simulink model "model"  (R2024b)
settings: Solver=ode1  StartTime=0.0  StopTime=10  FixedStep=0.0001  RelTol=1e-3
values from neighbouring files (symbols this model uses):
  a1 = c*a2    (= 810)    [init.m]
  a2 = c*a3    (= 270)    [init.m]
  a3 = c*a4    (= 90)    [init.m]
  a4 = c*10    (= 30)    [init.m]
  c1 = 50    [init.m]
  c2 = 1    [init.m]
  d = 100    [init.m]
  dis_gain = 30    [init.m]
  epsilon = 1    [init.m]
  i = 20    [init.m]
  k = 5    [init.m]
  mu = 0.9    [init.m]
  p = 400    [init.m]
  phi_frist = 0    [init.m]
  psi_frist = 0    [init.m]
  tau_p_max = 3000000    [init.m]
  theta_frist = 0    [init.m]
  umax = pi/2 - 0.01    (= 1.56079632679)    [init.m]
  w = wo    (= 50)    [init.m]
  wo = 50    [init.m]
  x_frist = 0    [init.m]
  y_frist = 0    [init.m]
  z_frist = 0    [init.m]
libraries: fod x36, slpidlib x6, simulink x1
(part 3 of 4)

== matlab function model/FO_SMC_ESO/Subsystem2/线性反馈 ==
  data: eta input; tau_1 output size=6; deta input; nu input; M_eta output; J output; J_inv output
function [tau_1,M_eta,J,J_inv] = fcn(eta,deta,nu)

m = 5.5;
    I_x = 0.12;
    I_y = 0.25;
    I_z = 0.2;
    V = m;
    g = 9.8;

    x_B = 0;
    y_B = 0;
    z_B = -0.01;

    X_du = -2.61;
    K_dp = -0.15;
    X_u = -2.47;
    K_P = -0.82;
    X_uu = -8.33;
    K_pp = -2.95;
    Y_dv = -5.56;
    M_dq = -0.26;
    Y_v = -3.54;
    M_q = -0.9;
    Y_vv = -10.82;
    M_qq = -3.687;
    Z_dw = -9.75;
    N_dr = -0.21;
    Z_w = -2.38;
    N_r = -0.45;
    Z_ww = -14.13;
    N_rr = -1.56;

    m_u = m - X_du;
    m_v = m - Y_dv;
    m_w = m - Z_dw;
    m_p = I_x - K_dp;
    m_q = I_y - M_dq;
    m_r = I_z - N_dr;

    m_u = m - X_du;
    m_v = m - Y_dv;
    m_w = m - Z_dw;
    m_p = I_x - K_dp;
    m_q = I_y - M_dq;
    m_r = I_z - N_dr;

    x = eta(1);
    y = eta(2);
    z = eta(3);
    phi = eta(4);
    theta = eta(5);
    psi = eta(6);

    J =  [cos(psi)*cos(theta) -sin(psi)*cos(phi)+sin(phi)*sin(theta)*cos(psi) sin(psi)*sin(phi)+sin(theta)*cos(psi)*cos(phi) 0 0 0;
         sin(psi)*cos(theta) cos(psi)*cos(phi)+sin(phi)*sin(theta)*sin(psi) -cos(psi)*sin(phi)+sin(theta)*sin(psi)*cos(phi) 0 0 0;
         -sin(theta) sin(phi)*cos(theta) cos(psi)*cos(theta) 0 0 0;
         0 0 0 1 sin(phi)*tan(theta) cos(phi)*tan(theta);
         0 0 0 0 cos(phi) -sin(phi);
         0 0 0 0 sin(phi)/cos(theta) cos(phi)/cos(theta)];

    J_inv = inv(J);

    u = nu(1);
    v = nu(2);
    w = nu(3);
    p = nu(4);
    q = nu(5);
    r = nu(6);

    
    dphi = deta(4);
    dtheta = deta(5);
    dpsi = deta(6);

    M = [m_u 0 0 0 0 0;
         0 m_v 0 0 0 0;
         0 0 m_w 0 0 0;
         0 0 0 m_p 0 0;
         0 0 0 0 m_q 0;
         0 0 0 0 0 m_r];

    C = [0 0 0 0 m_w*w -m_r*v;
         0 0 0 -m_w*w 0 m_u*u;
         0 0 0 m_v*v -m_u*u 0;
         0 m_w*w -m_v*v 0 m_r*r -m_q*q;
         -m_w*w 0 m_u*u -m_r*r 0 m_p*p;
         m_v*v -m_u*u 0 m_q*q -m_p*p 0];
    
    D = -[X_uu*abs(u) 0 0 0 0 0;
          0 Y_vv*abs(v) 0 0 0 0;
          0 0 Z_ww*abs(w) 0 0 0;
          0 0 0 K_pp*abs(p) 0 0;
          0 0 0 0 M_qq*abs(q) 0;
          0 0 0 0 0 N_rr*abs(r)];
    dJ = [
        % 第一行
        -sin(psi)*cos(theta)*dpsi - cos(psi)*sin(theta)*dtheta, ...
        (-cos(psi)*cos(phi) - sin(phi)*sin(theta)*sin(psi))*dpsi + ...
        (sin(phi)*cos(theta)*cos(psi))*dtheta + ...
        (sin(psi)*sin(phi) + cos(phi)*sin(theta)*cos(psi))*dphi, ...
        (cos(psi)*sin(phi) - sin(theta)*sin(psi)*cos(phi))*dpsi + ...
        (cos(psi)*cos(phi)*cos(theta))*dtheta + ...
        (sin(psi)*cos(phi) - sin(theta)*cos(psi)*sin(phi))*dphi, ...
        0, 0, 0;
        
        % 第二行
        cos(psi)*cos(theta)*dpsi - sin(psi)*sin(theta)*dtheta, ...
        (-sin(psi)*cos(phi) + sin(phi)*sin(theta)*cos(psi))*dpsi + ...
        (sin(phi)*cos(theta)*sin(psi))*dtheta + ...
        (-cos(psi)*sin(phi) + cos(phi)*sin(theta)*sin(psi))*dphi, ...
        (sin(psi)*sin(phi) + sin(theta)*cos(psi)*cos(phi))*dpsi + ...
        (sin(psi)*cos(phi)*cos(theta))*dtheta + ...
        (-cos(psi)*cos(phi) - sin(theta)*sin(psi)*sin(phi))*dphi, ...
        0, 0, 0;
        
        % 第三行
        -cos(theta)*dtheta, ...
        cos(phi)*cos(theta)*dphi - sin(phi)*sin(theta)*dtheta, ...
        -sin(psi)*cos(theta)*dpsi - cos(psi)*sin(theta)*dtheta, ...
        0, 0, 0;
        
        % 第四行
        0, 0, 0, ...
        0, ...
        cos(phi)*tan(theta)*dphi + sin(phi)*(1/cos(theta)^2)*dtheta, ...
        -sin(phi)*tan(theta)*dphi + cos(phi)*(1/cos(theta)^2)*dtheta;
        
        % 第五行
        0, 0, 0, ...
        0, ...
        -sin(phi)*dphi, ...
        -cos(phi)*dphi;
        
        % 第六行
        0, 0, 0, ...
        0, ...
        cos(phi)*(1/cos(theta))*dphi + sin(phi)*(sin(theta)/cos(theta)^2)*dtheta, ...
        -sin(phi)*(1/cos(theta))*dphi + cos(phi)*(sin(theta)/cos(theta)^2)*dtheta
    ];
    
    B = g*V;

    g_eta = [0;0;0;-z_B*B*cos(theta)*sin(phi);-z_B*B*sin(theta);0];

    M_eta = J_inv'*M*J_inv;
    C_eta = J_inv'*(C-M*J_inv*dJ)*J_inv;
    G_eta = J_inv'*g_eta;
    D_eta = J_inv'*D*J_inv;

tau_1 = J'*(C_eta*deta+D_eta*deta+G_eta);

== matlab function model/FO_SMC_ESO/LESO/Subsystem1/Subsystem6/MATLAB Function2 ==
  data: h input; dh output size=3; eta input; tau_0 input; wo input
function dh = fcn(h,eta,tau_0,wo)

e = eta-h(1);

b1 = 3*wo;
b2  = 3*wo^2;
b3 = wo^3;

dh = [h(2)+b1*e;
    h(3)+b2*e+tau_0;
    b3*e;
    ];

== matlab function model/tau_d/MATLAB Function ==
  data: t input; y output
function y = fcn(t)
    
y = [3*sin(t)*cos(t);3*sin(t)*cos(t);3*sin(t)*cos(t)];

== matlab function model/tau_d/MATLAB Function1 ==
  data: t input; y output
function y = fcn(t)
    
y = [3*sin(t)*cos(t);3*sin(t)*cos(t);3*sin(t)*cos(t)];

== matlab function model/FO_SMC_ESO/LESO/MATLAB Function3 ==
  data: M_eta input; tau_0 output; J_inv input; tau_c input
function tau_0 = fcn(M_eta,J_inv,tau_c)

tau_0 = inv(M_eta)*J_inv'*tau_c;

== matlab function model/FO_SMC_ESO/LESO/MATLAB Function4 ==
  data: J input; tau_2 output; M_eta input; h3 input
function tau_2 = fcn(J,M_eta,h3)

tau_2 = -J'*M_eta*h3;

== matlab function model/FO_SMC_ESO/LESO/Subsystem1/Subsystem1/MATLAB Function2 ==
  data: h input; dh output size=3; eta input; tau_0 input; wo input
function dh = fcn(h,eta,tau_0,wo)

e = eta-h(1);

b1 = 3*wo;
b2  = 3*wo^2;
b3 = wo^3;

dh = [h(2)+b1*e;
    h(3)+b2*e+tau_0;
    b3*e;
    ];

== matlab function model/FO_SMC_ESO/LESO/Subsystem1/Subsystem2/MATLAB Function2 ==
  data: h input; dh output size=3; eta input; tau_0 input; wo input
function dh = fcn(h,eta,tau_0,wo)

e = eta-h(1);

b1 = 3*wo;
b2  = 3*wo^2;
b3 = wo^3;

dh = [h(2)+b1*e;
    h(3)+b2*e+tau_0;
    b3*e;
    ];

== matlab function model/FO_SMC_ESO/LESO/Subsystem1/Subsystem3/MATLAB Function2 ==
  data: h input; dh output size=3; eta input; tau_0 input; wo input
function dh = fcn(h,eta,tau_0,wo)

e = eta-h(1);

b1 = 3*wo;
b2  = 3*wo^2;
b3 = wo^3;

dh = [h(2)+b1*e;
    h(3)+b2*e+tau_0;
    b3*e;
    ];

== matlab function model/FO_SMC_ESO/LESO/Subsystem1/Subsystem4/MATLAB Function2 ==
  data: h input; dh output size=3; eta input; tau_0 input; wo input
function dh = fcn(h,eta,tau_0,wo)

e = eta-h(1);

b1 = 3*wo;
b2  = 3*wo^2;
b3 = wo^3;

dh = [h(2)+b1*e;
    h(3)+b2*e+tau_0;
    b3*e;
    ];

== matlab function model/FO_SMC_ESO/Levant微分器/Subsystem1/MATLAB Function ==
  data: x input; z1_1 output; z1 input; z2 input; z3 input; z2_1 output; z3_1 output; z4 input; z4_1 output; a1 input; a2 input; a3 input; a4 input
function [z1_1,z2_1,z3_1,z4_1] = fcn(x,z1,z2,z3,z4,a1,a2,a3,a4)
    v1 = -a1*abs(z1-x)^(3/4)*sign(z1-x)+z2;
    z1_1 = v1;
    v2 = -a2*abs(z2-v1)^(2/3)*sign(z2-v1)+z3;
    z2_1 = v2;
    v3 = -a3*abs(z3-v2)^(1/2)*sign(z3-v2)+z4;
    z3_1 = v3;
    z4_1 = -a4*sign(z4-v3);
end

== matlab function model/FO_SMC_ESO/LESO/Subsystem1/Subsystem5/MATLAB Function2 ==
  data: h input; dh output size=3; eta input; tau_0 input; wo input
function dh = fcn(h,eta,tau_0,wo)

e = eta-h(1);

b1 = 3*wo;
b2  = 3*wo^2;
b3 = wo^3;

dh = [h(2)+b1*e;
    h(3)+b2*e+tau_0;
    b3*e;
    ];

== matlab function model/FO_SMC_ESO/Subsystem3/分数阶滑模 ==
  data: eta input; tau_3 output; deta input; D1 input; D2 input; c1 input; c2 input; eta_d input; deta_d input; ddeta_d input; k0 input; epsilon0 input; J input; M_eta input; ds output; h3 input
function [tau_3,ds] = fcn(eta,deta,D1,D2,c1,c2,eta_d,deta_d,ddeta_d,k0,epsilon0,J,M_eta,h3)
e = eta_d - eta;
de = deta_d - deta;

s = de + c1*e+c2*D1;

% ds =-( k0*s+epsilon0*sign(s));
k1 = 1;
epsilon1 = 0.01;

k = k0 + k1*abs(s);
epsilon = epsilon0 + epsilon1*abs(h3);

ds = -k.*s-epsilon.*(s./sqrt(s.^2+0.01^2));

tau_3 = J'*M_eta*(c1*de+c2*D2+ddeta_d-ds);

== matlab function model/FO_SMC_T/MATLAB Function1 ==
  data: eta input; nu output size=6; deta input
function nu = fcn(eta,deta)
    x = eta(1);
    y = eta(2);
    z = eta(3);
    phi = eta(4);
    theta = eta(5);
    psi = eta(6);

    J = [1 0 0 0 0 0;
         0 1 0 0 0 0;
         0 0 1 0 0 0;
         0 0 0 1 sin(phi)*tan(theta) cos(phi)*tan(theta);
         0 0 0 0 cos(phi) -sin(phi);
         0 0 0 0 sin(phi)/cos(theta) cos(phi)/cos(theta)];
    J_inv = inv(J);

nu = J_inv*deta;

== matlab function model/FO_SMC_T/Subsystem/Subsystem1/MATLAB Function ==
  data: x input; z1_1 output; z1 input; z2 input; z3 input; z2_1 output; z3_1 output; z4 input; z4_1 output; a1 input; a2 input; a3 input; a4 input
function [z1_1,z2_1,z3_1,z4_1] = fcn(x,z1,z2,z3,z4,a1,a2,a3,a4)
    v1 = -a1*abs(z1-x)^(3/4)*sign(z1-x)+z2;
    z1_1 = v1;
    v2 = -a2*abs(z2-v1)^(2/3)*sign(z2-v1)+z3;
    z2_1 = v2;
    v3 = -a3*abs(z3-v2)^(1/2)*sign(z3-v2)+z4;
    z3_1 = v3;
    z4_1 = -a4*sign(z4-v3);
end

== matlab function model/FO_SMC_T/Subsystem/Subsystem2/MATLAB Function ==
  data: x input; z1_1 output; z1 input; z2 input; z3 input; z2_1 output; z3_1 output; z4 input; z4_1 output; a1 input; a2 input; a3 input; a4 input
function [z1_1,z2_1,z3_1,z4_1] = fcn(x,z1,z2,z3,z4,a1,a2,a3,a4)
    v1 = -a1*abs(z1-x)^(3/4)*sign(z1-x)+z2;
    z1_1 = v1;
    v2 = -a2*abs(z2-v1)^(2/3)*sign(z2-v1)+z3;
    z2_1 = v2;
    v3 = -a3*abs(z3-v2)^(1/2)*sign(z3-v2)+z4;
    z3_1 = v3;
    z4_1 = -a4*sign(z4-v3);
end

== matlab function model/FO_SMC_T/Subsystem/Subsystem3/MATLAB Function ==
  data: x input; z1_1 output; z1 input; z2 input; z3 input; z2_1 output; z3_1 output; z4 input; z4_1 output; a1 input; a2 input; a3 input; a4 input
function [z1_1,z2_1,z3_1,z4_1] = fcn(x,z1,z2,z3,z4,a1,a2,a3,a4)
    v1 = -a1*abs(z1-x)^(3/4)*sign(z1-x)+z2;
    z1_1 = v1;
    v2 = -a2*abs(z2-v1)^(2/3)*sign(z2-v1)+z3;
    z2_1 = v2;
    v3 = -a3*abs(z3-v2)^(1/2)*sign(z3-v2)+z4;
    z3_1 = v3;
    z4_1 = -a4*sign(z4-v3);
end

== matlab function model/FO_SMC_T/MATLAB Function ==
  data: eta input; tau_p output size=6; eta_d input; deta input; deta_d input; ddeta_d input; nu input; D1 input; D2 input; k input; epsilon input; c1 input; c2 input
function tau_p   = fcn(eta,eta_d,deta,deta_d,ddeta_d,nu,D1,D2,k,epsilon,c1,c2)
    eta_e = eta - eta_d;
    deta_e = deta - deta_d;

    k = 150;
    c1 = 100;
    c2 = 10;
    epsilon = 5;

    s = eta_e + c1*eta_e + c2*D1;

    m = 5.5;
    I_x = 0.12;
    I_y = 0.25;
    I_z = 0.2;
    V = m;
    g = 9.8;

    x_B = 0;
    y_B = 0;
    z_B = -0.01;

    X_du = -2.61;
    K_dp = -0.15;
    X_u = -2.47;
    K_P = -0.82;
    X_uu = -8.33;
    K_pp = -2.95;
    Y_dv = -5.56;
    M_dq = -0.26;
    Y_v = -3.54;
    M_q = -0.9;
    Y_vv = -10.82;
    M_qq = -3.687;
    Z_dw = -9.75;
    N_dr = -0.21;
    Z_w = -2.38;
    N_r = -0.45;
    Z_ww = -14.13;
    N_rr = -1.56;

    m_u = m - X_du;
    m_v = m - Y_dv;
    m_w = m - Z_dw;
    m_p = I_x - K_dp;
    m_q = I_y - M_dq;
    m_r = I_z - N_dr;

    m_u = m - X_du;
    m_v = m - Y_dv;
    m_w = m - Z_dw;
    m_p = I_x - K_dp;
    m_q = I_y - M_dq;
    m_r = I_z - N_dr;

    x = eta(1);
    y = eta(2);
    z = eta(3);
    phi = eta(4);
    theta = eta(5);
    psi = eta(6);

    J = [1 0 0 0 0 0;
         0 1 0 0 0 0;
         0 0 1 0 0 0;
         0 0 0 1 sin(phi)*tan(theta) cos(phi)*tan(theta);
         0 0 0 0 cos(phi) -sin(phi);
         0 0 0 0 sin(phi)/cos(theta) cos(phi)/cos(theta)];
    J_inv = inv(J);

    u = nu(1);
    v = nu(2);
    w = nu(3);
    p = nu(4);
    q = nu(5);
    r = nu(6);

    
    dphi = deta(4);
    dtheta = deta(5);
    dpsi = deta(6);

    M = [m_u 0 0 0 0 0;
         0 m_v 0 0 0 0;
         0 0 m_w 0 0 0;
         0 0 0 m_p 0 0;
         0 0 0 0 m_q 0;
         0 0 0 0 0 m_r];

    C = [0 0 0 0 m_w*w -m_r*v;
         0 0 0 -m_w*w 0 m_u*u;
         0 0 0 m_v*v -m_u*u 0;
         0 m_w*w -m_v*v 0 m_r*r -m_q*q;
         -m_w*w 0 m_u*u -m_r*r 0 m_p*p;
         m_v*v -m_u*u 0 m_q*q -m_p*p 0];
    
    D = -[X_uu*abs(u) 0 0 0 0 0;
          0 Y_vv*abs(v) 0 0 0 0;
          0 0 Z_ww*abs(w) 0 0 0;
          0 0 0 K_pp*abs(p) 0 0;
          0 0 0 0 M_qq*abs(q) 0;
          0 0 0 0 0 N_rr*abs(r)];
    
    B = g*V;

    g_eta = [0;0;0;-z_B*B*cos(theta)*sin(phi);-z_B*B*sin(theta);0];

    

    dJ = [0 0 0 0 0 0;
         0 0 0 0 0 0;
         0 0 0 0 0 0;
         0 0 0 0 dphi*cos(phi)*tan(theta)+sin(phi)*dtheta/(cos(theta)*cos(theta)) -dphi*sin(phi)*tan(theta)+cos(phi)*dtheta/(cos(theta)*cos(theta));
         0 0 0 0 -dphi*sin(phi) -dphi*cos(phi);
         0 0 0 0 (dphi*cos(phi)*cos(theta)+dtheta*sin(phi)*sin(theta))/(cos(theta)*cos(theta)) (-dphi*sin(phi)*cos(theta)+dtheta*sin(theta)*cos(phi))/(cos(theta)*cos(theta))];

    M_ = J_inv'*M*J_inv;

    C_ = J_inv'*(C - M*J_inv*dJ)*J_inv;

    G_ = J_inv'*g_eta;

    D_ = J_inv' * D*J_inv;

    M_inv = inv(M_);
    
tau_p = J'*(C_*deta+D_*deta+G_) - J'*M_*(k*s + epsilon*sign(s) - ddeta_d + c1*deta_e + c2*D2);

== matlab function model/FO_SMC_T/Subsystem/Subsystem4/MATLAB Function ==
  data: x input; z1_1 output; z1 input; z2 input; z3 input; z2_1 output; z3_1 output; z4 input; z4_1 output; a1 input; a2 input; a3 input; a4 input
function [z1_1,z2_1,z3_1,z4_1] = fcn(x,z1,z2,z3,z4,a1,a2,a3,a4)
    v1 = -a1*abs(z1-x)^(3/4)*sign(z1-x)+z2;
    z1_1 = v1;
    v2 = -a2*abs(z2-v1)^(2/3)*sign(z2-v1)+z3;
    z2_1 = v2;
    v3 = -a3*abs(z3-v2)^(1/2)*sign(z3-v2)+z4;
    z3_1 = v3;
    z4_1 = -a4*sign(z4-v3);
end

== matlab function model/FO_SMC_T/Subsystem/Subsystem5/MATLAB Function ==
  data: x input; z1_1 output; z1 input; z2 input; z3 input; z2_1 output; z3_1 output; z4 input; z4_1 output; a1 input; a2 input; a3 input; a4 input
function [z1_1,z2_1,z3_1,z4_1] = fcn(x,z1,z2,z3,z4,a1,a2,a3,a4)
    v1 = -a1*abs(z1-x)^(3/4)*sign(z1-x)+z2;
    z1_1 = v1;
    v2 = -a2*abs(z2-v1)^(2/3)*sign(z2-v1)+z3;
    z2_1 = v2;
    v3 = -a3*abs(z3-v2)^(1/2)*sign(z3-v2)+z4;
    z3_1 = v3;
    z4_1 = -a4*sign(z4-v3);
end

== matlab function model/FO_SMC_T/Subsystem/Subsystem6/MATLAB Function ==
  data: x input; z1_1 output; z1 input; z2 input; z3 input; z2_1 output; z3_1 output; z4 input; z4_1 output; a1 input; a2 input; a3 input; a4 input
function [z1_1,z2_1,z3_1,z4_1] = fcn(x,z1,z2,z3,z4,a1,a2,a3,a4)
    v1 = -a1*abs(z1-x)^(3/4)*sign(z1-x)+z2;
    z1_1 = v1;
    v2 = -a2*abs(z2-v1)^(2/3)*sign(z2-v1)+z3;
    z2_1 = v2;
    v3 = -a3*abs(z3-v2)^(1/2)*sign(z3-v2)+z4;
    z3_1 = v3;
    z4_1 = -a4*sign(z4-v3);
end

== matlab function model/eta_d_y/MATLAB Function1 ==
  data: t input; y output
function y = fcn(t)
    
y = [0.12*pi*cos(0.04*pi*t);
    -0.12*pi*sin(0.04*pi*t);
    0.3];

== matlab function model/FO_SMC_T/Subsystem2/MATLAB Function6 ==
  data: x input; e output size=6; x_d input
function e  = fcn(x,x_d)

e = x - x_d;

== matlab function model/FO_SMC_ESO/Levant微分器/Subsystem2/MATLAB Function ==
  data: x input; z1_1 output; z1 input; z2 input; z3 input; z2_1 output; z3_1 output; z4 input; z4_1 output; a1 input; a2 input; a3 input; a4 input
function [z1_1,z2_1,z3_1,z4_1] = fcn(x,z1,z2,z3,z4,a1,a2,a3,a4)
    v1 = -a1*abs(z1-x)^(3/4)*sign(z1-x)+z2;
    z1_1 = v1;
    v2 = -a2*abs(z2-v1)^(2/3)*sign(z2-v1)+z3;
    z2_1 = v2;
    v3 = -a3*abs(z3-v2)^(1/2)*sign(z3-v2)+z4;
    z3_1 = v3;
    z4_1 = -a4*sign(z4-v3);
end

== matlab function model/eta_d_y/MATLAB Function2 ==
  data: t input; y output
function y = fcn(t)
    
y = [-0.0048*pi*pi*sin(0.04*pi*t);
    -0.0048*pi*pi*cos(0.04*pi*t);
    0];

== matlab function model/FO_SMC_ESO/Subsystem2/MATLAB Function1 ==
  data: eta input; nu output size=6; deta input
function nu = fcn(eta,deta)
    x = eta(1);
    y = eta(2);
    z = eta(3);
    phi = eta(4);
    theta = eta(5);
    psi = eta(6);

    J =  [cos(psi)*cos(theta) -sin(psi)*cos(phi)+sin(phi)*sin(theta)*cos(psi) sin(psi)*sin(phi)+sin(theta)*cos(psi)*cos(phi) 0 0 0;
         sin(psi)*cos(theta) cos(psi)*cos(phi)+sin(phi)*sin(theta)*sin(psi) -cos(psi)*sin(phi)+sin(theta)*sin(psi)*cos(phi) 0 0 0;
         -sin(theta) sin(phi)*cos(theta) cos(psi)*cos(theta) 0 0 0;
         0 0 0 1 sin(phi)*tan(theta) cos(phi)*tan(theta);
         0 0 0 0 cos(phi) -sin(phi);
         0 0 0 0 sin(phi)/cos(theta) cos(phi)/cos(theta)];
    J_inv = inv(J);

nu = J_inv*deta;

== matlab function model/系统3/MATLAB Function ==
  data: dnu output size=6*1; nu input; eta input; tau_p input; tau_d input; del input
function dnu = fcn(nu,eta,tau_p,tau_d,del)
    m = 5.5;
    I_x = 0.12;
    I_y = 0.25;
    I_z = 0.2;
    V = m;
    g = 9.8;

    x_B = 0;
    y_B = 0;
    z_B = -0.01;

    X_du = -2.61;
    K_dp = -0.15;
    X_u = -2.47;
    K_P = -0.82;
    X_uu = -8.33;
    K_pp = -2.95;
    Y_dv = -5.56;
    M_dq = -0.26;
    Y_v = -3.54;
    M_q = -0.9;
    Y_vv = -10.82;
    M_qq = -3.687;
    Z_dw = -9.75;
    N_dr = -0.21;
    Z_w = -2.38;
    N_r = -0.45;
    Z_ww = -14.13;
    N_rr = -1.56;

    m_u = m - X_du;
    m_v = m - Y_dv;
    m_w = m - Z_dw;
    m_p = I_x - K_dp;
    m_q = I_y - M_dq;
    m_r = I_z - N_dr;

    u = nu(1);
    v = nu(2);
    w = nu(3);
    p = nu(4);
    q = nu(5);
    r = nu(6);

    x = eta(1);
    y = eta(2);
    z = eta(3);
    phi = eta(4);
    theta = eta(5);
    psi = eta(6);

    M = [m_u 0 0 0 0 0;
         0 m_v 0 0 0 0;
         0 0 m_w 0 0 0;
         0 0 0 m_p 0 0;
         0 0 0 0 m_q 0;
         0 0 0 0 0 m_r];

    M = M+del*M;

    C = [0 0 0 0 m_w*w -m_r*v;
         0 0 0 -m_w*w 0 m_u*u;
         0 0 0 m_v*v -m_u*u 0;
         0 m_w*w -m_v*v 0 m_r*r -m_q*q;
         -m_w*w 0 m_u*u -m_r*r 0 m_p*p;
         m_v*v -m_u*u 0 m_q*q -m_p*p 0];

    C = C+del*C;
    
    D = -[X_uu*abs(u) 0 0 0 0 0;
          0 Y_vv*abs(v) 0 0 0 0;
          0 0 Z_ww*abs(w) 0 0 0;
          0 0 0 K_pp*abs(p) 0 0;
          0 0 0 0 M_qq*abs(q) 0;
          0 0 0 0 0 N_rr*abs(r)];

    D = D+del*D;
    
    B = g*V;

    g_eta = [0;0;0;-z_B*B*cos(theta)*sin(phi);-z_B*B*sin(theta);0];

    g_eta = g_eta+del*g_eta;

dnu = M\(tau_p + tau_d - C*nu - D*nu - g_eta);

== matlab function model/系统3/MATLAB Function1 ==
  data: eta input; deta output size=6*1; nv input
function deta = fcn(eta,nv)
    phi = eta(4);
    theta = eta(5);
    psi = eta(6);

    J =  [cos(psi)*cos(theta) -sin(psi)*cos(phi)+sin(phi)*sin(theta)*cos(psi) sin(psi)*sin(phi)+sin(theta)*cos(psi)*cos(phi) 0 0 0;
         sin(psi)*cos(theta) cos(psi)*cos(phi)+sin(phi)*sin(theta)*sin(psi) -cos(psi)*sin(phi)+sin(theta)*sin(psi)*cos(phi) 0 0 0;
         -sin(theta) sin(phi)*cos(theta) cos(psi)*cos(theta) 0 0 0;
         0 0 0 1 sin(phi)*tan(theta) cos(phi)*tan(theta);
         0 0 0 0 cos(phi) -sin(phi);
         0 0 0 0 sin(phi)/cos(theta) cos(phi)/cos(theta)];

deta = J*nv;

== matlab function model/系统1/MATLAB Function ==
  data: dnu output size=6*1; nu input; eta input; tau_p input; tau_d input; del input
function dnu = fcn(nu,eta,tau_p,tau_d,del)
    m = 5.5;
    I_x = 0.12;
    I_y = 0.25;
    I_z = 0.2;
    V = m;
    g = 9.8;

    x_B = 0;
    y_B = 0;
    z_B = -0.01;

    X_du = -2.61;
    K_dp = -0.15;
    X_u = -2.47;
    K_P = -0.82;
    X_uu = -8.33;
    K_pp = -2.95;
    Y_dv = -5.56;
    M_dq = -0.26;
    Y_v = -3.54;
    M_q = -0.9;
    Y_vv = -10.82;
    M_qq = -3.687;
    Z_dw = -9.75;
    N_dr = -0.21;
    Z_w = -2.38;
    N_r = -0.45;
    Z_ww = -14.13;
    N_rr = -1.56;

    m_u = m - X_du;
    m_v = m - Y_dv;
    m_w = m - Z_dw;
    m_p = I_x - K_dp;
    m_q = I_y - M_dq;
    m_r = I_z - N_dr;

    u = nu(1);
    v = nu(2);
    w = nu(3);
    p = nu(4);
    q = nu(5);
    r = nu(6);

    x = eta(1);
    y = eta(2);
    z = eta(3);
    phi = eta(4);
    theta = eta(5);
    psi = eta(6);

    M = [m_u 0 0 0 0 0;
         0 m_v 0 0 0 0;
         0 0 m_w 0 0 0;
         0 0 0 m_p 0 0;
         0 0 0 0 m_q 0;
         0 0 0 0 0 m_r];

    M = M+del*M;

    C = [0 0 0 0 m_w*w -m_r*v;
         0 0 0 -m_w*w 0 m_u*u;
         0 0 0 m_v*v -m_u*u 0;
         0 m_w*w -m_v*v 0 m_r*r -m_q*q;
         -m_w*w 0 m_u*u -m_r*r 0 m_p*p;
         m_v*v -m_u*u 0 m_q*q -m_p*p 0];

    C = C+del*C;
    
    D = -[X_uu*abs(u) 0 0 0 0 0;
          0 Y_vv*abs(v) 0 0 0 0;
          0 0 Z_ww*abs(w) 0 0 0;
          0 0 0 K_pp*abs(p) 0 0;
          0 0 0 0 M_qq*abs(q) 0;
          0 0 0 0 0 N_rr*abs(r)];

    D = D+del*D;
    
    B = g*V;

    g_eta = [0;0;0;-z_B*B*cos(theta)*sin(phi);-z_B*B*sin(theta);0];

    g_eta = g_eta+del*g_eta;

dnu = M\(tau_p + tau_d - C*nu - D*nu - g_eta);

== matlab function model/系统1/MATLAB Function1 ==
  data: eta input; deta output size=6*1; nv input
function deta = fcn(eta,nv)
    phi = eta(4);
    theta = eta(5);
    psi = eta(6);

    J =  [cos(psi)*cos(theta) -sin(psi)*cos(phi)+sin(phi)*sin(theta)*cos(psi) sin(psi)*sin(phi)+sin(theta)*cos(psi)*cos(phi) 0 0 0;
         sin(psi)*cos(theta) cos(psi)*cos(phi)+sin(phi)*sin(theta)*sin(psi) -cos(psi)*sin(phi)+sin(theta)*sin(psi)*cos(phi) 0 0 0;
         -sin(theta) sin(phi)*cos(theta) cos(psi)*cos(theta) 0 0 0;
         0 0 0 1 sin(phi)*tan(theta) cos(phi)*tan(theta);
         0 0 0 0 cos(phi) -sin(phi);
         0 0 0 0 sin(phi)/cos(theta) cos(phi)/cos(theta)];

deta = J*nv;

== matlab function model/系统4/MATLAB Function ==
  data: dnu output size=6*1; nu input; eta input; tau_p input; tau_d input; del input
function dnu = fcn(nu,eta,tau_p,tau_d,del)
    m = 5.5;
    I_x = 0.12;
    I_y = 0.25;
    I_z = 0.2;
    V = m;
    g = 9.8;

    x_B = 0;
    y_B = 0;
    z_B = -0.01;

    X_du = -2.61;
    K_dp = -0.15;
    X_u = -2.47;
    K_P = -0.82;
    X_uu = -8.33;
    K_pp = -2.95;
    Y_dv = -5.56;
    M_dq = -0.26;
    Y_v = -3.54;
    M_q = -0.9;
    Y_vv = -10.82;
    M_qq = -3.687;
    Z_dw = -9.75;
    N_dr = -0.21;
    Z_w = -2.38;
    N_r = -0.45;
    Z_ww = -14.13;
    N_rr = -1.56;

    m_u = m - X_du;
    m_v = m - Y_dv;
    m_w = m - Z_dw;
    m_p = I_x - K_dp;
    m_q = I_y - M_dq;
    m_r = I_z - N_dr;

    u = nu(1);
    v = nu(2);
    w = nu(3);
    p = nu(4);
    q = nu(5);
    r = nu(6);

    x = eta(1);
    y = eta(2);
    z = eta(3);
    phi = eta(4);
    theta = eta(5);
    psi = eta(6);

    M = [m_u 0 0 0 0 0;
         0 m_v 0 0 0 0;
         0 0 m_w 0 0 0;
         0 0 0 m_p 0 0;
         0 0 0 0 m_q 0;
         0 0 0 0 0 m_r];

    M = M+del*M;

    C = [0 0 0 0 m_w*w -m_r*v;
         0 0 0 -m_w*w 0 m_u*u;
         0 0 0 m_v*v -m_u*u 0;
         0 m_w*w -m_v*v 0 m_r*r -m_q*q;
         -m_w*w 0 m_u*u -m_r*r 0 m_p*p;
         m_v*v -m_u*u 0 m_q*q -m_p*p 0];

    C = C+del*C;
    
    D = -[X_uu*abs(u) 0 0 0 0 0;
          0 Y_vv*abs(v) 0 0 0 0;
          0 0 Z_ww*abs(w) 0 0 0;
          0 0 0 K_pp*abs(p) 0 0;
          0 0 0 0 M_qq*abs(q) 0;
          0 0 0 0 0 N_rr*abs(r)];

    D = D+del*D;
    
    B = g*V;

    g_eta = [0;0;0;-z_B*B*cos(theta)*sin(phi);-z_B*B*sin(theta);0];

    g_eta = g_eta+del*g_eta;

dnu = M\(tau_p + tau_d - C*nu - D*nu - g_eta);

== matlab function model/系统4/MATLAB Function1 ==
  data: eta input; deta output size=6*1; nv input
function deta = fcn(eta,nv)
    phi = eta(4);
    theta = eta(5);
    psi = eta(6);

    J =  [cos(psi)*cos(theta) -sin(psi)*cos(phi)+sin(phi)*sin(theta)*cos(psi) sin(psi)*sin(phi)+sin(theta)*cos(psi)*cos(phi) 0 0 0;
         sin(psi)*cos(theta) cos(psi)*cos(phi)+sin(phi)*sin(theta)*sin(psi) -cos(psi)*sin(phi)+sin(theta)*sin(psi)*cos(phi) 0 0 0;
         -sin(theta) sin(phi)*cos(theta) cos(psi)*cos(theta) 0 0 0;
         0 0 0 1 sin(phi)*tan(theta) cos(phi)*tan(theta);
         0 0 0 0 cos(phi) -sin(phi);
         0 0 0 0 sin(phi)/cos(theta) cos(phi)/cos(theta)];

deta = J*nv;

== matlab function model/系统2/MATLAB Function ==
  data: dnu output size=6*1; nu input; eta input; tau_p input; tau_d input; del input
function dnu = fcn(nu,eta,tau_p,tau_d,del)
    m = 5.5;
    I_x = 0.12;
    I_y = 0.25;
    I_z = 0.2;
    V = m;
    g = 9.8;

    x_B = 0;
    y_B = 0;
    z_B = -0.01;

    X_du = -2.61;
    K_dp = -0.15;
    X_u = -2.47;
    K_P = -0.82;
    X_uu = -8.33;
    K_pp = -2.95;
    Y_dv = -5.56;
    M_dq = -0.26;
    Y_v = -3.54;
    M_q = -0.9;
    Y_vv = -10.82;
    M_qq = -3.687;
    Z_dw = -9.75;
    N_dr = -0.21;
    Z_w = -2.38;
    N_r = -0.45;
    Z_ww = -14.13;
    N_rr = -1.56;

    m_u = m - X_du;
    m_v = m - Y_dv;
    m_w = m - Z_dw;
    m_p = I_x - K_dp;
    m_q = I_y - M_dq;
    m_r = I_z - N_dr;

    u = nu(1);
    v = nu(2);
    w = nu(3);
    p = nu(4);
    q = nu(5);
    r = nu(6);

    x = eta(1);
    y = eta(2);
    z = eta(3);
    phi = eta(4);
    theta = eta(5);
    psi = eta(6);

    M = [m_u 0 0 0 0 0;
         0 m_v 0 0 0 0;
         0 0 m_w 0 0 0;
         0 0 0 m_p 0 0;
         0 0 0 0 m_q 0;
         0 0 0 0 0 m_r];

    M = M+del*M;

    C = [0 0 0 0 m_w*w -m_r*v;
         0 0 0 -m_w*w 0 m_u*u;
         0 0 0 m_v*v -m_u*u 0;
         0 m_w*w -m_v*v 0 m_r*r -m_q*q;
         -m_w*w 0 m_u*u -m_r*r 0 m_p*p;
         m_v*v -m_u*u 0 m_q*q -m_p*p 0];

    C = C+del*C;
    
    D = -[X_uu*abs(u) 0 0 0 0 0;
          0 Y_vv*abs(v) 0 0 0 0;
          0 0 Z_ww*abs(w) 0 0 0;
          0 0 0 K_pp*abs(p) 0 0;
          0 0 0 0 M_qq*abs(q) 0;
          0 0 0 0 0 N_rr*abs(r)];

    D = D+del*D;
    
    B = g*V;

    g_eta = [0;0;0;-z_B*B*cos(theta)*sin(phi);-z_B*B*sin(theta);0];

    g_eta = g_eta+del*g_eta;

dnu = M\(tau_p + tau_d - C*nu - D*nu - g_eta);

== matlab function model/系统2/MATLAB Function1 ==
  data: eta input; deta output size=6*1; nv input
function deta = fcn(eta,nv)
    phi = eta(4);
    theta = eta(5);
    psi = eta(6);

    J =  [cos(psi)*cos(theta) -sin(psi)*cos(phi)+sin(phi)*sin(theta)*cos(psi) sin(psi)*sin(phi)+sin(theta)*cos(psi)*cos(phi) 0 0 0;
         sin(psi)*cos(theta) cos(psi)*cos(phi)+sin(phi)*sin(theta)*sin(psi) -cos(psi)*sin(phi)+sin(theta)*sin(psi)*cos(phi) 0 0 0;
         -sin(theta) sin(phi)*cos(theta) cos(psi)*cos(theta) 0 0 0;
         0 0 0 1 sin(phi)*tan(theta) cos(phi)*tan(theta);
         0 0 0 0 cos(phi) -sin(phi);
         0 0 0 0 sin(phi)/cos(theta) cos(phi)/cos(theta)];

deta = J*nv;

== matlab function model/eta_d_y1/MATLAB Function ==
  data: t input; y output
function y = fcn(t)
    
y = [3;4;5];

== matlab function model/eta_d_y1/MATLAB Function1 ==
  data: t input; y output
function y = fcn(t)
    
y = [0;
    0;
    0];

== matlab function model/eta_d_y1/MATLAB Function2 ==
  data: t input; y output
function y = fcn(t)
    
y = [0;
    0;
    0];

== matlab function model/FO_SMC/MATLAB Function ==
  data: eta input; tau_p output size=6; eta_d input; deta input; deta_d input; ddeta_d input; nu input; D1 input; D2 input; c1 input; c2 input; k input; epsilon input
function tau_p   = fcn(eta,eta_d,deta,deta_d,ddeta_d,nu,D1,D2,c1,c2,k,epsilon)
    a1 = c1;
    a2 = c2;
    % b = 0.01;
    % F = 30;
    xi = epsilon;

    eta_e = eta - eta_d;
    deta_e = deta - deta_d;

    s = eta_e + a1*eta_e + a2*D1;

    m = 5.5;
    I_x = 0.12;
    I_y = 0.25;
    I_z = 0.2;
    V = m;
    g = 9.8;

    x_B = 0;
    y_B = 0;
    z_B = -0.01;

    X_du = -2.61;
    K_dp = -0.15;
    X_u = -2.47;
    K_P = -0.82;
    X_uu = -8.33;
    K_pp = -2.95;
    Y_dv = -5.56;
    M_dq = -0.26;
    Y_v = -3.54;
    M_q = -0.9;
    Y_vv = -10.82;
    M_qq = -3.687;
    Z_dw = -9.75;
    N_dr = -0.21;
    Z_w = -2.38;
    N_r = -0.45;
    Z_ww = -14.13;
    N_rr = -1.56;

    m_u = m - X_du;
    m_v = m - Y_dv;
    m_w = m - Z_dw;
    m_p = I_x - K_dp;
    m_q = I_y - M_dq;
    m_r = I_z - N_dr;

    m_u = m - X_du;
    m_v = m - Y_dv;
    m_w = m - Z_dw;
    m_p = I_x - K_dp;
    m_q = I_y - M_dq;
    m_r = I_z - N_dr;

    x = eta(1);
    y = eta(2);
    z = eta(3);
    phi = eta(4);
    theta = eta(5);
    psi = eta(6);

    J =  [cos(psi)*cos(theta) -sin(psi)*cos(phi)+sin(phi)*sin(theta)*cos(psi) sin(psi)*sin(phi)+sin(theta)*cos(psi)*cos(phi) 0 0 0;
         sin(psi)*cos(theta) cos(psi)*cos(phi)+sin(phi)*sin(theta)*sin(psi) -cos(psi)*sin(phi)+sin(theta)*sin(psi)*cos(phi) 0 0 0;
         -sin(theta) sin(phi)*cos(theta) cos(psi)*cos(theta) 0 0 0;
         0 0 0 1 sin(phi)*tan(theta) cos(phi)*tan(theta);
         0 0 0 0 cos(phi) -sin(phi);
         0 0 0 0 sin(phi)/cos(theta) cos(phi)/cos(theta)];
    J_inv = inv(J);

    u = nu(1);
    v = nu(2);
    w = nu(3);
    p = nu(4);
    q = nu(5);
    r = nu(6);

    
    dphi = deta(4);
    dtheta = deta(5);
    dpsi = deta(6);

    M = [m_u 0 0 0 0 0;
         0 m_v 0 0 0 0;
         0 0 m_w 0 0 0;
         0 0 0 m_p 0 0;
         0 0 0 0 m_q 0;
         0 0 0 0 0 m_r];

    C = [0 0 0 0 m_w*w -m_r*v;
         0 0 0 -m_w*w 0 m_u*u;
         0 0 0 m_v*v -m_u*u 0;
         0 m_w*w -m_v*v 0 m_r*r -m_q*q;
         -m_w*w 0 m_u*u -m_r*r 0 m_p*p;
         m_v*v -m_u*u 0 m_q*q -m_p*p 0];
    
    D = -[X_uu*abs(u) 0 0 0 0 0;
          0 Y_vv*abs(v) 0 0 0 0;
          0 0 Z_ww*abs(w) 0 0 0;
          0 0 0 K_pp*abs(p) 0 0;
          0 0 0 0 M_qq*abs(q) 0;
          0 0 0 0 0 N_rr*abs(r)];
    
    B = g*V;

    g_eta = [0;0;0;-z_B*B*cos(theta)*sin(phi);-z_B*B*sin(theta);0];

    

    dJ = [
        % 第一行
        -sin(psi)*cos(theta)*dpsi - cos(psi)*sin(theta)*dtheta, ...
        (-cos(psi)*cos(phi) - sin(phi)*sin(theta)*sin(psi))*dpsi + ...
        (sin(phi)*cos(theta)*cos(psi))*dtheta + ...
        (sin(psi)*sin(phi) + cos(phi)*sin(theta)*cos(psi))*dphi, ...
        (cos(psi)*sin(phi) - sin(theta)*sin(psi)*cos(phi))*dpsi + ...
        (cos(psi)*cos(phi)*cos(theta))*dtheta + ...
        (sin(psi)*cos(phi) - sin(theta)*cos(psi)*sin(phi))*dphi, ...
        0, 0, 0;
        
        % 第二行
        cos(psi)*cos(theta)*dpsi - sin(psi)*sin(theta)*dtheta, ...
        (-sin(psi)*cos(phi) + sin(phi)*sin(theta)*cos(psi))*dpsi + ...
        (sin(phi)*cos(theta)*sin(psi))*dtheta + ...
        (-cos(psi)*sin(phi) + cos(phi)*sin(theta)*sin(psi))*dphi, ...
        (sin(psi)*sin(phi) + sin(theta)*cos(psi)*cos(phi))*dpsi + ...
        (sin(psi)*cos(phi)*cos(theta))*dtheta + ...
        (-cos(psi)*cos(phi) - sin(theta)*sin(psi)*sin(phi))*dphi, ...
        0, 0, 0;
        
        % 第三行
        -cos(theta)*dtheta, ...
        cos(phi)*cos(theta)*dphi - sin(phi)*sin(theta)*dtheta, ...
        -sin(psi)*cos(theta)*dpsi - cos(psi)*sin(theta)*dtheta, ...
        0, 0, 0;
        
        % 第四行
        0, 0, 0, ...
        0, ...
        cos(phi)*tan(theta)*dphi + sin(phi)*(1/cos(theta)^2)*dtheta, ...
        -sin(phi)*tan(theta)*dphi + cos(phi)*(1/cos(theta)^2)*dtheta;
        
        % 第五行
        0, 0, 0, ...
        0, ...
        -sin(phi)*dphi, ...
        -cos(phi)*dphi;
        
        % 第六行
        0, 0, 0, ...
        0, ...
        cos(phi)*(1/cos(theta))*dphi + sin(phi)*(sin(theta)/cos(theta)^2)*dtheta, ...
        -sin(phi)*(1/cos(theta))*dphi + cos(phi)*(sin(theta)/cos(theta)^2)*dtheta
    ];

    M_ = J_inv'*M*J_inv;

    C_ = J_inv'*(C - M*J_inv*dJ)*J_inv;

    G_ = J_inv'*g_eta;

    D_ = J_inv' * D*J_inv;

    M_inv = inv(M_);
    
tau_p = J'*(C_*deta+D_*deta+G_) - J'*M_*(k*s + xi*sign(s) - ddeta_d + a1*deta_e + a2*D2);

== matlab function model/FO_SMC/MATLAB Function1 ==
  data: eta input; nu output size=6; deta input
function nu = fcn(eta,deta)
    x = eta(1);
    y = eta(2);
    z = eta(3);
    phi = eta(4);
    theta = eta(5);
    psi = eta(6);

    J =  [cos(psi)*cos(theta) -sin(psi)*cos(phi)+sin(phi)*sin(theta)*cos(psi) sin(psi)*sin(phi)+sin(theta)*cos(psi)*cos(phi) 0 0 0;
         sin(psi)*cos(theta) cos(psi)*cos(phi)+sin(phi)*sin(theta)*sin(psi) -cos(psi)*sin(phi)+sin(theta)*sin(psi)*cos(phi) 0 0 0;
         -sin(theta) sin(phi)*cos(theta) cos(psi)*cos(theta) 0 0 0;
         0 0 0 1 sin(phi)*tan(theta) cos(phi)*tan(theta);
         0 0 0 0 cos(phi) -sin(phi);
         0 0 0 0 sin(phi)/cos(theta) cos(phi)/cos(theta)];
    J_inv = inv(J);

nu = J_inv*deta;

== matlab function model/FO_SMC/Subsystem/Subsystem1/MATLAB Function ==
  data: x input; z1_1 output; z1 input; z2 input; z3 input; z2_1 output; z3_1 output; z4 input; z4_1 output; a1 input; a2 input; a3 input; a4 input
function [z1_1,z2_1,z3_1,z4_1] = fcn(x,z1,z2,z3,z4,a1,a2,a3,a4)
    v1 = -a1*abs(z1-x)^(3/4)*sign(z1-x)+z2;
    z1_1 = v1;
    v2 = -a2*abs(z2-v1)^(2/3)*sign(z2-v1)+z3;
    z2_1 = v2;
    v3 = -a3*abs(z3-v2)^(1/2)*sign(z3-v2)+z4;
    z3_1 = v3;
    z4_1 = -a4*sign(z4-v3);
end

== matlab function model/FO_SMC/Subsystem/Subsystem2/MATLAB Function ==
  data: x input; z1_1 output; z1 input; z2 input; z3 input; z2_1 output; z3_1 output; z4 input; z4_1 output; a1 input; a2 input; a3 input; a4 input
function [z1_1,z2_1,z3_1,z4_1] = fcn(x,z1,z2,z3,z4,a1,a2,a3,a4)
    v1 = -a1*abs(z1-x)^(3/4)*sign(z1-x)+z2;
    z1_1 = v1;
    v2 = -a2*abs(z2-v1)^(2/3)*sign(z2-v1)+z3;
    z2_1 = v2;
    v3 = -a3*abs(z3-v2)^(1/2)*sign(z3-v2)+z4;
    z3_1 = v3;
    z4_1 = -a4*sign(z4-v3);
end

== matlab function model/FO_SMC/Subsystem/Subsystem3/MATLAB Function ==
  data: x input; z1_1 output; z1 input; z2 input; z3 input; z2_1 output; z3_1 output; z4 input; z4_1 output; a1 input; a2 input; a3 input; a4 input
function [z1_1,z2_1,z3_1,z4_1] = fcn(x,z1,z2,z3,z4,a1,a2,a3,a4)
    v1 = -a1*abs(z1-x)^(3/4)*sign(z1-x)+z2;
    z1_1 = v1;
    v2 = -a2*abs(z2-v1)^(2/3)*sign(z2-v1)+z3;
    z2_1 = v2;
    v3 = -a3*abs(z3-v2)^(1/2)*sign(z3-v2)+z4;
    z3_1 = v3;
    z4_1 = -a4*sign(z4-v3);
end

== matlab function model/FO_SMC_ESO/Levant微分器/Subsystem3/MATLAB Function ==
  data: x input; z1_1 output; z1 input; z2 input; z3 input; z2_1 output; z3_1 output; z4 input; z4_1 output; a1 input; a2 input; a3 input; a4 input
function [z1_1,z2_1,z3_1,z4_1] = fcn(x,z1,z2,z3,z4,a1,a2,a3,a4)
    v1 = -a1*abs(z1-x)^(3/4)*sign(z1-x)+z2;
    z1_1 = v1;
    v2 = -a2*abs(z2-v1)^(2/3)*sign(z2-v1)+z3;
    z2_1 = v2;
    v3 = -a3*abs(z3-v2)^(1/2)*sign(z3-v2)+z4;
    z3_1 = v3;
    z4_1 = -a4*sign(z4-v3);
end

== matlab function model/FO_SMC/Subsystem/Subsystem4/MATLAB Function ==
  data: x input; z1_1 output; z1 input; z2 input; z3 input; z2_1 output; z3_1 output; z4 input; z4_1 output; a1 input; a2 input; a3 input; a4 input
function [z1_1,z2_1,z3_1,z4_1] = fcn(x,z1,z2,z3,z4,a1,a2,a3,a4)
    v1 = -a1*abs(z1-x)^(3/4)*sign(z1-x)+z2;
    z1_1 = v1;
    v2 = -a2*abs(z2-v1)^(2/3)*sign(z2-v1)+z3;
    z2_1 = v2;
    v3 = -a3*abs(z3-v2)^(1/2)*sign(z3-v2)+z4;
    z3_1 = v3;
    z4_1 = -a4*sign(z4-v3);
end

== matlab function model/FO_SMC/Subsystem/Subsystem5/MATLAB Function ==
  data: x input; z1_1 output; z1 input; z2 input; z3 input; z2_1 output; z3_1 output; z4 input; z4_1 output; a1 input; a2 input; a3 input; a4 input
function [z1_1,z2_1,z3_1,z4_1] = fcn(x,z1,z2,z3,z4,a1,a2,a3,a4)
    v1 = -a1*abs(z1-x)^(3/4)*sign(z1-x)+z2;
    z1_1 = v1;
    v2 = -a2*abs(z2-v1)^(2/3)*sign(z2-v1)+z3;
    z2_1 = v2;
    v3 = -a3*abs(z3-v2)^(1/2)*sign(z3-v2)+z4;
    z3_1 = v3;
    z4_1 = -a4*sign(z4-v3);
end

== matlab function model/FO_SMC/Subsystem/Subsystem6/MATLAB Function ==
  data: x input; z1_1 output; z1 input; z2 input; z3 input; z2_1 output; z3_1 output; z4 input; z4_1 output; a1 input; a2 input; a3 input; a4 input
function [z1_1,z2_1,z3_1,z4_1] = fcn(x,z1,z2,z3,z4,a1,a2,a3,a4)
    v1 = -a1*abs(z1-x)^(3/4)*sign(z1-x)+z2;
    z1_1 = v1;
    v2 = -a2*abs(z2-v1)^(2/3)*sign(z2-v1)+z3;
    z2_1 = v2;
    v3 = -a3*abs(z3-v2)^(1/2)*sign(z3-v2)+z4;
    z3_1 = v3;
    z4_1 = -a4*sign(z4-v3);
end

== matlab function model/ADRC/控制器/6路levant微分器/Subsystem1/MATLAB Function ==
  data: x input; z1_1 output; z1 input; z2 input; z3 input; z2_1 output; z3_1 output; z4 input; z4_1 output
function [z1_1,z2_1,z3_1,z4_1] = fcn(x,z1,z2,z3,z4)
    
    a1 = 20;
    a2 = 20;
    a3 = 20;
    a4 = 20;

    v1 = -a1*abs(z1-x)^(3/4)*sign(z1-x)+z2;
    z1_1 = v1;
    v2 = -a2*abs(z2-v1)^(2/3)*sign(z2-v1)+z3;
    z2_1 = v2;
    v3 = -a3*abs(z3-v2)^(1/2)*sign(z3-v2)+z4;
    z3_1 = v3;
    z4_1 = -a4*sign(z4-v3);
end

== matlab function model/ADRC/控制器/6路levant微分器/Subsystem2/MATLAB Function ==
  data: x input; z1_1 output; z1 input; z2 input; z3 input; z2_1 output; z3_1 output; z4 input; z4_1 output
function [z1_1,z2_1,z3_1,z4_1] = fcn(x,z1,z2,z3,z4)
    
    a1 = 20;
    a2 = 20;
    a3 = 20;
    a4 = 20;

    v1 = -a1*abs(z1-x)^(3/4)*sign(z1-x)+z2;
    z1_1 = v1;
    v2 = -a2*abs(z2-v1)^(2/3)*sign(z2-v1)+z3;
    z2_1 = v2;
    v3 = -a3*abs(z3-v2)^(1/2)*sign(z3-v2)+z4;
    z3_1 = v3;
    z4_1 = -a4*sign(z4-v3);
end

== matlab function model/ADRC/控制器/6路levant微分器/Subsystem3/MATLAB Function ==
  data: x input; z1_1 output; z1 input; z2 input; z3 input; z2_1 output; z3_1 output; z4 input; z4_1 output
function [z1_1,z2_1,z3_1,z4_1] = fcn(x,z1,z2,z3,z4)
    
    a1 = 20;
    a2 = 20;
    a3 = 20;
    a4 = 20;

    v1 = -a1*abs(z1-x)^(3/4)*sign(z1-x)+z2;
    z1_1 = v1;
    v2 = -a2*abs(z2-v1)^(2/3)*sign(z2-v1)+z3;
    z2_1 = v2;
    v3 = -a3*abs(z3-v2)^(1/2)*sign(z3-v2)+z4;
    z3_1 = v3;
    z4_1 = -a4*sign(z4-v3);
end

== matlab function model/ADRC/控制器/6路levant微分器/Subsystem4/MATLAB Function ==
  data: x input; z1_1 output; z1 input; z2 input; z3 input; z2_1 output; z3_1 output; z4 input; z4_1 output
function [z1_1,z2_1,z3_1,z4_1] = fcn(x,z1,z2,z3,z4)
    
    a1 = 20;
    a2 = 20;
    a3 = 20;
    a4 = 20;

    v1 = -a1*abs(z1-x)^(3/4)*sign(z1-x)+z2;
    z1_1 = v1;
    v2 = -a2*abs(z2-v1)^(2/3)*sign(z2-v1)+z3;
    z2_1 = v2;
    v3 = -a3*abs(z3-v2)^(1/2)*sign(z3-v2)+z4;
    z3_1 = v3;
    z4_1 = -a4*sign(z4-v3);
end

== matlab function model/ADRC/控制器/6路levant微分器/Subsystem5/MATLAB Function ==
  data: x input; z1_1 output; z1 input; z2 input; z3 input; z2_1 output; z3_1 output; z4 input; z4_1 output
function [z1_1,z2_1,z3_1,z4_1] = fcn(x,z1,z2,z3,z4)
    
    a1 = 20;
    a2 = 20;
    a3 = 20;
    a4 = 20;

    v1 = -a1*abs(z1-x)^(3/4)*sign(z1-x)+z2;
    z1_1 = v1;
    v2 = -a2*abs(z2-v1)^(2/3)*sign(z2-v1)+z3;
    z2_1 = v2;
    v3 = -a3*abs(z3-v2)^(1/2)*sign(z3-v2)+z4;
    z3_1 = v3;
    z4_1 = -a4*sign(z4-v3);
end

== matlab function model/ADRC/控制器/6路levant微分器/Subsystem6/MATLAB Function ==
  data: x input; z1_1 output; z1 input; z2 input; z3 input; z2_1 output; z3_1 output; z4 input; z4_1 output
function [z1_1,z2_1,z3_1,z4_1] = fcn(x,z1,z2,z3,z4)
    
    a1 = 20;
    a2 = 20;
    a3 = 20;
    a4 = 20;

    v1 = -a1*abs(z1-x)^(3/4)*sign(z1-x)+z2;
    z1_1 = v1;
    v2 = -a2*abs(z2-v1)^(2/3)*sign(z2-v1)+z3;
    z2_1 = v2;
    v3 = -a3*abs(z3-v2)^(1/2)*sign(z3-v2)+z4;
    z3_1 = v3;
    z4_1 = -a4*sign(z4-v3);
end

== matlab function model/FO_SMC/Subsystem2/MATLAB Function6 ==
  data: x input; e output size=6; x_d input
function e  = fcn(x,x_d)

e = x - x_d;

== matlab function model/ADRC/控制器/MATLAB Function ==
  data: r input; dr input; ddr input; tau_p output; x1 input; x2 input; x3 input; wo input; eta input; u0 output
function [tau_p,u0] = fcn(r,dr,ddr,x1,x2,x3,wo,eta)
    
    m = 5.5;
    I_x = 0.12;
    I_y = 0.25;
    I_z = 0.2;
    V = m;
    g = 9.8;

    x_B = 0;
    y_B = 0;
    z_B = -0.01;

    X_du = -2.61;
    K_dp = -0.15;
    X_u = -2.47;
    K_P = -0.82;
    X_uu = -8.33;
    K_pp = -2.95;
    Y_dv = -5.56;
    M_dq = -0.26;
    Y_v = -3.54;
    M_q = -0.9;
    Y_vv = -10.82;
    M_qq = -3.687;
    Z_dw = -9.75;
    N_dr = -0.21;
    Z_w = -2.38;
    N_r = -0.45;
    Z_ww = -14.13;
    N_rr = -1.56;

    m_u = m - X_du;
    m_v = m - Y_dv;
    m_w = m - Z_dw;
    m_p = I_x - K_dp;
    m_q = I_y - M_dq;
    m_r = I_z - N_dr;

    m_u = m - X_du;
    m_v = m - Y_dv;
    m_w = m - Z_dw;
    m_p = I_x - K_dp;
    m_q = I_y - M_dq;
    m_r = I_z - N_dr;    

    x = eta(1);
    y = eta(2);
    z = eta(3);
    phi = eta(4);
    theta = eta(5);
    psi = eta(6);

    J =  [cos(psi)*cos(theta) -sin(psi)*cos(phi)+sin(phi)*sin(theta)*cos(psi) sin(psi)*sin(phi)+sin(theta)*cos(psi)*cos(phi) 0 0 0;
         sin(psi)*cos(theta) cos(psi)*cos(phi)+sin(phi)*sin(theta)*sin(psi) -cos(psi)*sin(phi)+sin(theta)*sin(psi)*cos(phi) 0 0 0;
         -sin(theta) sin(phi)*cos(theta) cos(psi)*cos(theta) 0 0 0;
         0 0 0 1 sin(phi)*tan(theta) cos(phi)*tan(theta);
         0 0 0 0 cos(phi) -sin(phi);
         0 0 0 0 sin(phi)/cos(theta) cos(phi)/cos(theta)];
    
    J_inv = inv(J);

    M = [m_u 0 0 0 0 0;
         0 m_v 0 0 0 0;
         0 0 m_w 0 0 0;
         0 0 0 m_p 0 0;
         0 0 0 0 m_q 0;
         0 0 0 0 0 m_r];

    M_ = J_inv'*M*J_inv;

    tau_p = J'*M_*(wo^2*(r-x1)+2*wo*(dr-x2)+ddr-x3);

    u0 = wo^2*(r-x1)+2*wo*(dr-x2)+ddr-x3;
end

== matlab function model/SMC/MATLAB Function ==
  data: eta input; tau_p output size=6; eta_d input; deta input; deta_d input; ddeta_d input; nu input; c1 input; k input; epsilon input
function tau_p   = fcn(eta,eta_d,deta,deta_d,ddeta_d,nu,c1,k,epsilon)
    a1 = c1;
    % b = 0.01;
    % F = 30;
    xi = epsilon;

    eta_e = eta - eta_d;
    deta_e = deta - deta_d;

    s = eta_e + a1*eta_e ;

    m = 5.5;
    I_x = 0.12;
    I_y = 0.25;
    I_z = 0.2;
    V = m;
    g = 9.8;

    x_B = 0;
    y_B = 0;
    z_B = -0.01;

    X_du = -2.61;
    K_dp = -0.15;
    X_u = -2.47;
    K_P = -0.82;
    X_uu = -8.33;
    K_pp = -2.95;
    Y_dv = -5.56;
    M_dq = -0.26;
    Y_v = -3.54;
    M_q = -0.9;
    Y_vv = -10.82;
    M_qq = -3.687;
    Z_dw = -9.75;
    N_dr = -0.21;
    Z_w = -2.38;
    N_r = -0.45;
    Z_ww = -14.13;
    N_rr = -1.56;

    m_u = m - X_du;
    m_v = m - Y_dv;
    m_w = m - Z_dw;
    m_p = I_x - K_dp;
    m_q = I_y - M_dq;
    m_r = I_z - N_dr;

    m_u = m - X_du;
    m_v = m - Y_dv;
    m_w = m - Z_dw;
    m_p = I_x - K_dp;
    m_q = I_y - M_dq;
    m_r = I_z - N_dr;

    x = eta(1);
    y = eta(2);
    z = eta(3);
    phi = eta(4);
    theta = eta(5);
    psi = eta(6);

    J =  [cos(psi)*cos(theta) -sin(psi)*cos(phi)+sin(phi)*sin(theta)*cos(psi) sin(psi)*sin(phi)+sin(theta)*cos(psi)*cos(phi) 0 0 0;
         sin(psi)*cos(theta) cos(psi)*cos(phi)+sin(phi)*sin(theta)*sin(psi) -cos(psi)*sin(phi)+sin(theta)*sin(psi)*cos(phi) 0 0 0;
         -sin(theta) sin(phi)*cos(theta) cos(psi)*cos(theta) 0 0 0;
         0 0 0 1 sin(phi)*tan(theta) cos(phi)*tan(theta);
         0 0 0 0 cos(phi) -sin(phi);
         0 0 0 0 sin(phi)/cos(theta) cos(phi)/cos(theta)];
    J_inv = inv(J);

    u = nu(1);
    v = nu(2);
    w = nu(3);
    p = nu(4);
    q = nu(5);
    r = nu(6);

    
    dphi = deta(4);
    dtheta = deta(5);
    dpsi = deta(6);

    M = [m_u 0 0 0 0 0;
         0 m_v 0 0 0 0;
         0 0 m_w 0 0 0;
         0 0 0 m_p 0 0;
         0 0 0 0 m_q 0;
         0 0 0 0 0 m_r];

    C = [0 0 0 0 m_w*w -m_r*v;
         0 0 0 -m_w*w 0 m_u*u;
         0 0 0 m_v*v -m_u*u 0;
         0 m_w*w -m_v*v 0 m_r*r -m_q*q;
         -m_w*w 0 m_u*u -m_r*r 0 m_p*p;
         m_v*v -m_u*u 0 m_q*q -m_p*p 0];
    
    D = -[X_uu*abs(u) 0 0 0 0 0;
          0 Y_vv*abs(v) 0 0 0 0;
          0 0 Z_ww*abs(w) 0 0 0;
          0 0 0 K_pp*abs(p) 0 0;
          0 0 0 0 M_qq*abs(q) 0;
          0 0 0 0 0 N_rr*abs(r)];
    
    B = g*V;

    g_eta = [0;0;0;-z_B*B*cos(theta)*sin(phi);-z_B*B*sin(theta);0];

    

    dJ = [
        % 第一行
        -sin(psi)*cos(theta)*dpsi - cos(psi)*sin(theta)*dtheta, ...
        (-cos(psi)*cos(phi) - sin(phi)*sin(theta)*sin(psi))*dpsi + ...
        (sin(phi)*cos(theta)*cos(psi))*dtheta + ...
        (sin(psi)*sin(phi) + cos(phi)*sin(theta)*cos(psi))*dphi, ...
        (cos(psi)*sin(phi) - sin(theta)*sin(psi)*cos(phi))*dpsi + ...
        (cos(psi)*cos(phi)*cos(theta))*dtheta + ...
        (sin(psi)*cos(phi) - sin(theta)*cos(psi)*sin(phi))*dphi, ...
        0, 0, 0;
        
        % 第二行
        cos(psi)*cos(theta)*dpsi - sin(psi)*sin(theta)*dtheta, ...
        (-sin(psi)*cos(phi) + sin(phi)*sin(theta)*cos(psi))*dpsi + ...
        (sin(phi)*cos(theta)*sin(psi))*dtheta + ...
        (-cos(psi)*sin(phi) + cos(phi)*sin(theta)*sin(psi))*dphi, ...
        (sin(psi)*sin(phi) + sin(theta)*cos(psi)*cos(phi))*dpsi + ...
        (sin(psi)*cos(phi)*cos(theta))*dtheta + ...
        (-cos(psi)*cos(phi) - sin(theta)*sin(psi)*sin(phi))*dphi, ...
        0, 0, 0;
        
        % 第三行
        -cos(theta)*dtheta, ...
        cos(phi)*cos(theta)*dphi - sin(phi)*sin(theta)*dtheta, ...
        -sin(psi)*cos(theta)*dpsi - cos(psi)*sin(theta)*dtheta, ...
        0, 0, 0;
        
        % 第四行
        0, 0, 0, ...
        0, ...
        cos(phi)*tan(theta)*dphi + sin(phi)*(1/cos(theta)^2)*dtheta, ...
        -sin(phi)*tan(theta)*dphi + cos(phi)*(1/cos(theta)^2)*dtheta;
        
        % 第五行
        0, 0, 0, ...
        0, ...
        -sin(phi)*dphi, ...
        -cos(phi)*dphi;
        
        % 第六行
        0, 0, 0, ...
        0, ...
        cos(phi)*(1/cos(theta))*dphi + sin(phi)*(sin(theta)/cos(theta)^2)*dtheta, ...
        -sin(phi)*(1/cos(theta))*dphi + cos(phi)*(sin(theta)/cos(theta)^2)*dtheta
    ];

    M_ = J_inv'*M*J_inv;

    C_ = J_inv'*(C - M*J_inv*dJ)*J_inv;

    G_ = J_inv'*g_eta;

    D_ = J_inv' * D*J_inv;

    M_inv = inv(M_);
    
tau_p = J'*(C_*deta+D_*deta+G_) - J'*M_*(k*s + xi*sign(s) - ddeta_d + a1*deta_e );
% format(tau_p);

== matlab function model/FO_SMC_ESO/Levant微分器/Subsystem5/MATLAB Function ==
  data: x input; z1_1 output; z1 input; z2 input; z3 input; z2_1 output; z3_1 output; z4 input; z4_1 output; a1 input; a2 input; a3 input; a4 input
function [z1_1,z2_1,z3_1,z4_1] = fcn(x,z1,z2,z3,z4,a1,a2,a3,a4)
    v1 = -a1*abs(z1-x)^(3/4)*sign(z1-x)+z2;
    z1_1 = v1;
    v2 = -a2*abs(z2-v1)^(2/3)*sign(z2-v1)+z3;
    z2_1 = v2;
    v3 = -a3*abs(z3-v2)^(1/2)*sign(z3-v2)+z4;
    z3_1 = v3;
    z4_1 = -a4*sign(z4-v3);
end

== matlab function model/SMC/MATLAB Function1 ==
  data: eta input; nu output size=6; deta input
function nu = fcn(eta,deta)
    x = eta(1);
    y = eta(2);
    z = eta(3);
    phi = eta(4);
    theta = eta(5);
    psi = eta(6);

    J =  [cos(psi)*cos(theta) -sin(psi)*cos(phi)+sin(phi)*sin(theta)*cos(psi) sin(psi)*sin(phi)+sin(theta)*cos(psi)*cos(phi) 0 0 0;
         sin(psi)*cos(theta) cos(psi)*cos(phi)+sin(phi)*sin(theta)*sin(psi) -cos(psi)*sin(phi)+sin(theta)*sin(psi)*cos(phi) 0 0 0;
         -sin(theta) sin(phi)*cos(theta) cos(psi)*cos(theta) 0 0 0;
         0 0 0 1 sin(phi)*tan(theta) cos(phi)*tan(theta);
         0 0 0 0 cos(phi) -sin(phi);
         0 0 0 0 sin(phi)/cos(theta) cos(phi)/cos(theta)];
    J_inv = inv(J);

nu = J_inv*deta;

== matlab function model/SMC/Subsystem/Subsystem1/MATLAB Function ==
  data: x input; z1_1 output; z1 input; z2 input; z3 input; z2_1 output; z3_1 output; z4 input; z4_1 output; a1 input; a2 input; a3 input; a4 input
function [z1_1,z2_1,z3_1,z4_1] = fcn(x,z1,z2,z3,z4,a1,a2,a3,a4)
    v1 = -a1*abs(z1-x)^(3/4)*sign(z1-x)+z2;
    z1_1 = v1;
    v2 = -a2*abs(z2-v1)^(2/3)*sign(z2-v1)+z3;
    z2_1 = v2;
    v3 = -a3*abs(z3-v2)^(1/2)*sign(z3-v2)+z4;
    z3_1 = v3;
    z4_1 = -a4*sign(z4-v3);
end

== matlab function model/SMC/Subsystem/Subsystem2/MATLAB Function ==
  data: x input; z1_1 output; z1 input; z2 input; z3 input; z2_1 output; z3_1 output; z4 input; z4_1 output; a1 input; a2 input; a3 input; a4 input
function [z1_1,z2_1,z3_1,z4_1] = fcn(x,z1,z2,z3,z4,a1,a2,a3,a4)
    v1 = -a1*abs(z1-x)^(3/4)*sign(z1-x)+z2;
    z1_1 = v1;
    v2 = -a2*abs(z2-v1)^(2/3)*sign(z2-v1)+z3;
    z2_1 = v2;
    v3 = -a3*abs(z3-v2)^(1/2)*sign(z3-v2)+z4;
    z3_1 = v3;
    z4_1 = -a4*sign(z4-v3);
end

== matlab function model/FO_SMC_ESO/Levant微分器/Subsystem4/MATLAB Function ==
  data: x input; z1_1 output; z1 input; z2 input; z3 input; z2_1 output; z3_1 output; z4 input; z4_1 output; a1 input; a2 input; a3 input; a4 input
function [z1_1,z2_1,z3_1,z4_1] = fcn(x,z1,z2,z3,z4,a1,a2,a3,a4)
    v1 = -a1*abs(z1-x)^(3/4)*sign(z1-x)+z2;
    z1_1 = v1;
    v2 = -a2*abs(z2-v1)^(2/3)*sign(z2-v1)+z3;
    z2_1 = v2;
    v3 = -a3*abs(z3-v2)^(1/2)*sign(z3-v2)+z4;
    z3_1 = v3;
    z4_1 = -a4*sign(z4-v3);
end

== matlab function model/SMC/Subsystem/Subsystem3/MATLAB Function ==
  data: x input; z1_1 output; z1 input; z2 input; z3 input; z2_1 output; z3_1 output; z4 input; z4_1 output; a1 input; a2 input; a3 input; a4 input
function [z1_1,z2_1,z3_1,z4_1] = fcn(x,z1,z2,z3,z4,a1,a2,a3,a4)
    v1 = -a1*abs(z1-x)^(3/4)*sign(z1-x)+z2;
    z1_1 = v1;
    v2 = -a2*abs(z2-v1)^(2/3)*sign(z2-v1)+z3;
    z2_1 = v2;
    v3 = -a3*abs(z3-v2)^(1/2)*sign(z3-v2)+z4;
    z3_1 = v3;
    z4_1 = -a4*sign(z4-v3);
end

== matlab function model/SMC/Subsystem/Subsystem4/MATLAB Function ==
  data: x input; z1_1 output; z1 input; z2 input; z3 input; z2_1 output; z3_1 output; z4 input; z4_1 output; a1 input; a2 input; a3 input; a4 input
function [z1_1,z2_1,z3_1,z4_1] = fcn(x,z1,z2,z3,z4,a1,a2,a3,a4)
    v1 = -a1*abs(z1-x)^(3/4)*sign(z1-x)+z2;
    z1_1 = v1;
    v2 = -a2*abs(z2-v1)^(2/3)*sign(z2-v1)+z3;
    z2_1 = v2;
    v3 = -a3*abs(z3-v2)^(1/2)*sign(z3-v2)+z4;
    z3_1 = v3;
    z4_1 = -a4*sign(z4-v3);
end

== matlab function model/SMC/Subsystem/Subsystem5/MATLAB Function ==
  data: x input; z1_1 output; z1 input; z2 input; z3 input; z2_1 output; z3_1 output; z4 input; z4_1 output; a1 input; a2 input; a3 input; a4 input
function [z1_1,z2_1,z3_1,z4_1] = fcn(x,z1,z2,z3,z4,a1,a2,a3,a4)
    v1 = -a1*abs(z1-x)^(3/4)*sign(z1-x)+z2;
    z1_1 = v1;
    v2 = -a2*abs(z2-v1)^(2/3)*sign(z2-v1)+z3;
    z2_1 = v2;
    v3 = -a3*abs(z3-v2)^(1/2)*sign(z3-v2)+z4;
    z3_1 = v3;
    z4_1 = -a4*sign(z4-v3);
end
